simulink model "SI4_Roll_Dynamics"  (R2019b)
settings: Solver=VariableStepAuto  StartTime=0.0  StopTime=10.0  RelTol=1e-3
values from neighbouring files (symbols this model uses):
  c_0 = 1/(m*(h^2))    [C2_Preliminary_Controller_Design.m]    (also in D1_Preliminary_Controller_Design.m = 26.7908045386; D2_Controller_Design.m = 26.7908045386; D3_PL_Controller_Design.m = 79.9725508614; D4_DPDZ_Controller_Design.m = 79.9725508614)
  c_1 = m*g*h    [C2_Preliminary_Controller_Design.m]    (also in D1_Preliminary_Controller_Design.m = 3.790584; D2_Controller_Design.m = 3.790584; D3_PL_Controller_Design.m = 1.26984564; D4_DPDZ_Controller_Design.m = 1.26984564)
  c_2 = m * a * h * sine_lambda/ b    [C2_Preliminary_Controller_Design.m]    (also in D1_Preliminary_Controller_Design.m; D2_Controller_Design.m; D3_PL_Controller_Design.m; D4_DPDZ_Controller_Design.m)
  c_3 = m * a * c * g * sine_lambda/ b    [C2_Preliminary_Controller_Design.m]    (also in D1_Preliminary_Controller_Design.m; D2_Controller_Design.m; D3_PL_Controller_Design.m; D4_DPDZ_Controller_Design.m)
  c_4 = m * h * sine_lambda/ b    [C2_Preliminary_Controller_Design.m]    (also in D1_Preliminary_Controller_Design.m; D2_Controller_Design.m; D3_PL_Controller_Design.m; D4_DPDZ_Controller_Design.m)
  c_5 = h * sine_lambda/ b    [C2_Preliminary_Controller_Design.m]    (also in D1_Preliminary_Controller_Design.m; D2_Controller_Design.m; D3_PL_Controller_Design.m; D4_DPDZ_Controller_Design.m)
settings Model: Creator=Conor  LastModifiedBy=Conor
settings DataIOCC: SaveOutput=off  SignalLogging=off  DSMLogging=off  SaveTime=off  ReturnWorkspaceOutputs=off
settings SFSimCC: CustomCodeUndefinedFunction=UseInterfaceOnly

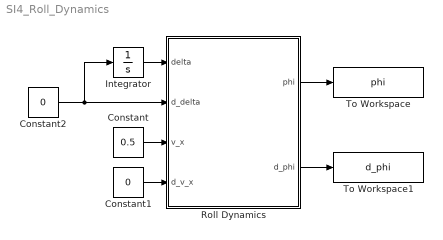
== system SI4_Roll_Dynamics ==
  Constant : Constant  Value=0.5
  Constant1 : Constant  Value=0
  Constant2 : Constant  Value=0
  Integrator : Integrator
  Roll Dynamics : Subsystem
  To Workspace : ToWorkspace  VariableName=phi  SampleTime=-1
  To Workspace1 : ToWorkspace  VariableName=d_phi  SampleTime=-1
  wires:
  Constant/1 -> Roll Dynamics/3(v_x)
  Constant1/1 -> Roll Dynamics/4(d_v_x)
  Constant2/1 -> Integrator/1, Roll Dynamics/2(d_delta)
  Roll Dynamics/1(phi) -> To Workspace/1
  Roll Dynamics/2(d_phi) -> To Workspace1/1
  Integrator/1 -> Roll Dynamics/1(delta)

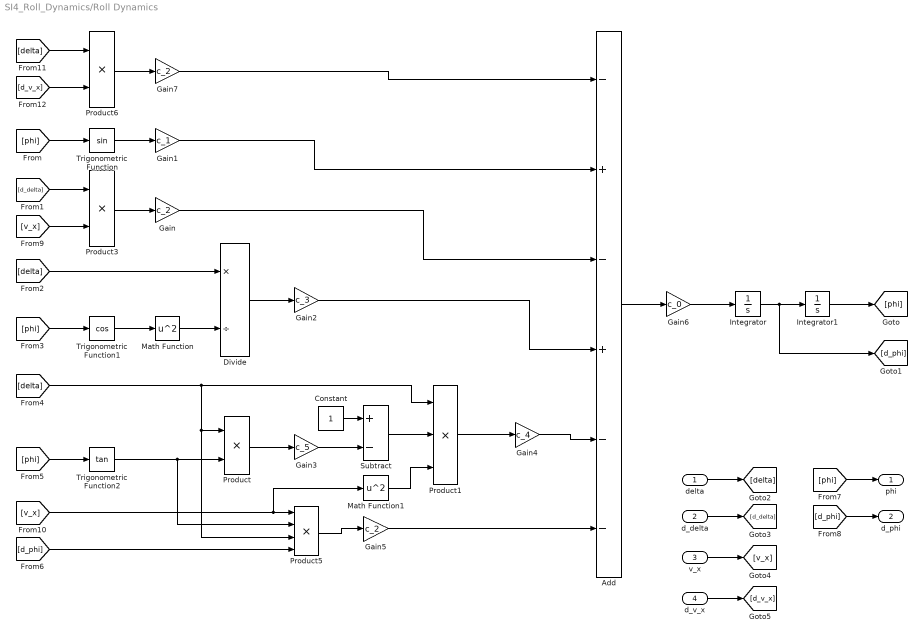
== system SI4_Roll_Dynamics/Roll Dynamics ==
  delta : Inport
  d_delta : Inport  Port=2
  v_x : Inport  Port=3
  d_v_x : Inport  Port=4
  Add : Sum  Inputs=-+-+--
  Constant : Constant
  Divide : Product  Inputs=*/
  Gain : Gain  Gain=c_2
  Gain1 : Gain  Gain=c_1
  Gain2 : Gain  Gain=c_3
  Gain3 : Gain  Gain=c_5
  Gain4 : Gain  Gain=c_4
  Gain5 : Gain  Gain=c_2
  Gain6 : Gain  Gain=c_0
  Gain7 : Gain  Gain=c_2
  Integrator : Integrator
  Integrator1 : Integrator
  Math Function : Math  Operator=square  SaturateOnIntegerOverflow=on
  Math Function1 : Math  Operator=square  SaturateOnIntegerOverflow=on
  Product : Product
  Product1 : Product  Inputs=3
  Product3 : Product
  Product5 : Product  Inputs=4
  Product6 : Product
  Subtract : Sum  Inputs=+-
  Trigonometric Function : Trigonometry
  Trigonometric Function1 : Trigonometry  Operator=cos
  Trigonometric Function2 : Trigonometry  Operator=tan
  phi : Outport  VectorParamsAs1DForOutWhenUnconnected=off
  d_phi : Outport  Port=2  VectorParamsAs1DForOutWhenUnconnected=off
  wires:
  Product/1 -> Gain3/1
  Gain2/1 -> Add/4
  Math Function/1 -> Divide/2
  Constant/1 -> Subtract/1
  Trigonometric Function/1 -> Gain1/1
  Gain6/1 -> Integrator/1
  [delta] -> Product5/3, Product/1, Product1/1
  Trigonometric Function2/1 -> Product5/2, Product/2
  [delta] -> Divide/1
  Gain4/1 -> Add/5
  Gain5/1 -> Add/6
  Integrator/1 -> Integrator1/1, [d_phi]
  Add/1 -> Gain6/1
  Integrator1/1 -> [phi]
  Subtract/1 -> Product1/2
  Gain/1 -> Add/3
  [phi] -> Trigonometric Function/1
  Divide/1 -> Gain2/1
  [phi] -> Trigonometric Function2/1
  [d_phi] -> Product5/4
  Trigonometric Function1/1 -> Math Function/1
  [phi] -> Trigonometric Function1/1
  Gain1/1 -> Add/2
  Gain3/1 -> Subtract/2
  [phi] -> phi/1
  [d_phi] -> d_phi/1
  delta/1 -> [delta]
  d_delta/1 -> [d_delta]
  Product3/1 -> Gain/1
  [d_delta] -> Product3/1
  [v_x] -> Product3/2
  Product1/1 -> Gain4/1
  Math Function1/1 -> Product1/3
  Product5/1 -> Gain5/1
  [v_x] -> Math Function1/1, Product5/1
  v_x/1 -> [v_x]
  d_v_x/1 -> [d_v_x]
  [delta] -> Product6/1
  [d_v_x] -> Product6/2
  Product6/1 -> Gain7/1
  Gain7/1 -> Add/1
